simulink model "projekatSimulink"  (R2023b)
settings: Solver=VariableStepAuto  StartTime=0.0  StopTime=10.0  RelTol=1e-3
values from neighbouring files (symbols this model uses):
  A = [0 1 0 0 0; a21 a22 a23 a24 0; 0 0 0 1 0; a41 a42 a43 a44 a45; 0 0 0 a54 a55]    [projekatMatlab.m]
  a21 = k/(5*m)    (= 4000)    [projekatMatlab.m]
  a22 = b/(5*m)    (= 0.75)    [projekatMatlab.m]
  a23 = -k/(5*m)    (= -4000)    [projekatMatlab.m]
  a24 = -b/(5*m)    (= -0.75)    [projekatMatlab.m]
  a41 = -k/Mt    (= -61538.4615385)    [projekatMatlab.m]
  a42 = -b/Mt    (= -11.5384615385)    [projekatMatlab.m]
  a43 = k/Mt    (= 61538.4615385)    [projekatMatlab.m]
  a44 = -(Bp+b)/Mt    (= -13.8461538462)    [projekatMatlab.m]
  a45 = Ap/Mt    (= 0.000230769230769)    [projekatMatlab.m]
  a54 = -4*Be*Ap/Vt    (= -3900000000)    [projekatMatlab.m]
  a55 = -(Ctp+Kc)*4*Be/Vt    (= -2.6)    [projekatMatlab.m]
  b = 150    [projekatMatlab.m]
  B = [0; 0; 0; 0; b51]    [projekatMatlab.m]
  b51 = Kq*4*Be*Kt/(Vt*r*R*Kf)    (= 95766666.6667)    [projekatMatlab.m]
  C = [1 0 0 0 0]    [projekatMatlab.m]
  k = 8e5    (= 800000)    [projekatMatlab.m]
libraries: slpidlib x1
settings Model: Creator=Mi-Store  LastModifiedBy=Mi-Store

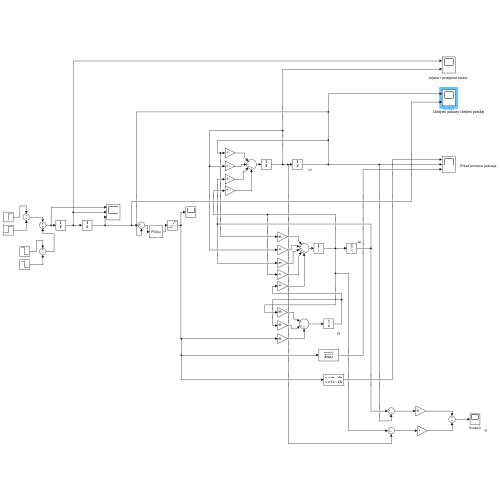
[thumbnail: Simulink's stored preview of the top-level diagram]
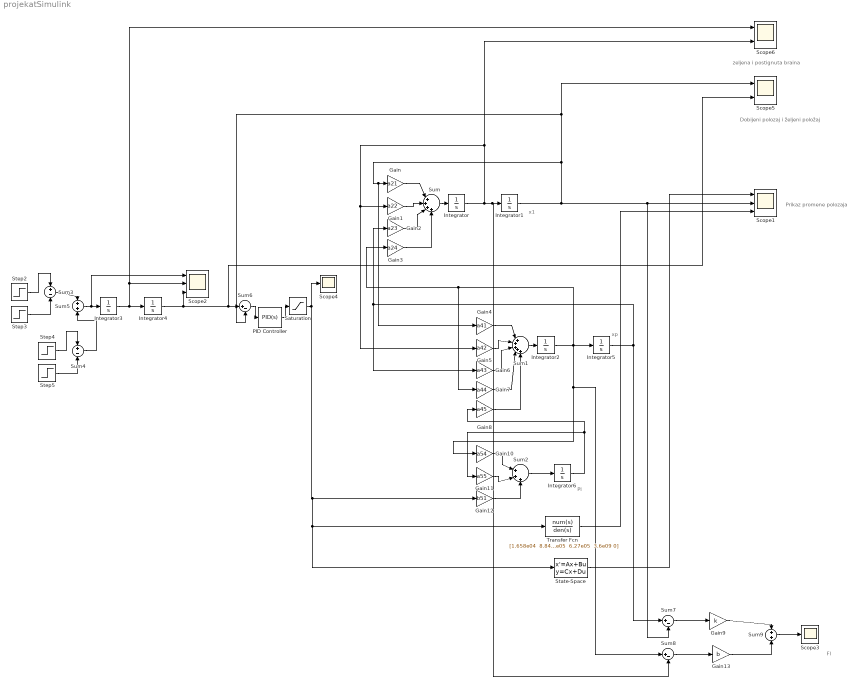
== system projekatSimulink ==
  note: zeljena i postignuta braina
  note: Dobijeni polozaj i željeni položaj
  note: Prikaz promene polozaja
  note: Fl
  note: Pl
  note: xp
  note: x1
  Gain : Gain  Gain=a21
  Gain1 : Gain  Gain=a22
  Gain10 : Gain  Gain=a54
  Gain11 : Gain  Gain=a55
  Gain12 : Gain  Gain=b51
  Gain13 : Gain  Gain=b
  Gain2 : Gain  Gain=a23
  Gain3 : Gain  Gain=a24
  Gain4 : Gain  Gain=a41
  Gain5 : Gain  Gain=a42
  Gain6 : Gain  Gain=a43
  Gain7 : Gain  Gain=a44
  Gain8 : Gain  Gain=a45
  Gain9 : Gain  Gain=k
  Integrator{,1..6} (7 alike) : Integrator
  PID Controller : slpidlib/PID Controller  Controller=PID  Form=Parallel  TimeDomain=Continuous-time  UseExternalTs=off  SampleTime=-1  IntegratorMethod=Forward Euler  FilterMethod=Forward Euler  ControllerParametersSource=internal  P=180  I=10  UseKiTs=on  D=0  N=100  UseFilter=on  TunerSelectOption=Transfer Function Based (PID Tuner App)  InitialConditionSource=internal  InitialConditionForIntegrator=0  InitialConditionForFilter=0  DifferentiatorICPrevScaledInput=0  ExternalReset=none  TrackingMode=off  Kt=1  LimitOutput=off  SatLimitsSource=internal  UpperSaturationLimit=inf  LowerSaturationLimit=-inf  LinearizeAsGain=on  AntiWindupMode=none  Kb=1  LimitIntegrator=off  UpperIntegratorSaturationLimit=inf  LowerIntegratorSaturationLimit=-inf  POutMin=[]  POutMax=[]  IOutMin=[]  IOutMax=[]  DOutMin=[]  DOutMax=[]  NOutMin=[]  NOutMax=[]  SumOutMin=[]  SumOutMax=[]  SaturationOutMin=[]  SaturationOutMax=[]  PParamMin=[]  PParamMax=[]  IParamMin=[]  IParamMax=[]  DParamMin=[]  DParamMax=[]  NParamMin=[]  NParamMax=[]  KbParamMin=[]  KbParamMax=[]  KtParamMin=[]  KtParamMax=[]  KbOutMin=[]  KbOutMax=[]  KtOutMin=[]  KtOutMax=[]  IntegratorOutMin=[]  IntegratorOutMax=[]  FilterOutMin=[]  FilterOutMax=[]  SumI1OutMin=[]  SumI1OutMax=[]  SumI2OutMin=[]  SumI2OutMax=[]  SumI3OutMin=[]  SumI3OutMax=[]  SumI4OutMin=[]  SumI4OutMax=[]  SumDOutMin=[]  SumDOutMax=[]  DifferentiatorOutMin=[]  DifferentiatorOutMax=[]  FilterDiffOutCoefMin=[]  FilterDiffOutCoefMax=[]  ReciprocalOutMin=[]  ReciprocalOutMax=[]  SumDenOutMin=[]  SumDenOutMax=[]  SumNumOutMin=[]  SumNumOutMax=[]  DivideOutMin=[]  DivideOutMax=[]  UdiffTsProdOutMin=[]  UdiffTsProdOutMax=[]  NTsProdOutMin=[]  NTsProdOutMax=[]  UintegralTsProdOutMin=[]  UintegralTsProdOutMax=[]  UngainTsProdOutMin=[]  UngainTsProdOutMax=[]  ClampingZeroOutDataTypeStr=Inherit: Inherit via back propagation  ClampingZeroOutMin=[]  ClampingZeroOutMax=[]  FilterDenConstantOutDataTypeStr=Inherit: Inherit via back propagation  FilterDenConstantOutMin=[]  FilterDenConstantOutMax=[]  PCopyOutDataTypeStr=Inherit: Inherit via back propagation  PCopyOutMin=[]  PCopyOutMax=[]  NCopyOutDataTypeStr=Inherit: Inherit via back propagation  NCopyOutMin=[]  NCopyOutMax=[]  IntegratorContinuousStateAttributes=''  IntegratorStateMustResolveToSignalObject=off  IntegratorRTWStateStorageClass=Auto  FilterContinuousStateAttributes=''  FilterStateMustResolveToSignalObject=off  FilterRTWStateStorageClass=Auto  ParallelPVariant=InternalParameters  IdealPVariant=Disabled  IVariant=InternalParameters  DVariant=InternalParameters  IntegratorVariant=Continuous  SatVariant=Disabled  AWVariant=Passthrough  PCopyVariant=Disabled  TRVariant=Disabled  FdbkBlocksVariant=Forward  IdealPFdbkVariant=Disabled  SatFdbkVariant=Disabled  DerivativeFilterVariant=ContFilter  NVariant=InternalParameters  NCopyVariant=Disabled  FilterICVariant=InternalICsFilter  IntegratorICVariant=InternalICs  ExternalResetVariant=Disabled  TRSumVariant=Passthrough  SumFdbkVariant=Disabled  SumVariant=Sum_PID  TsampFilterVariant=InternalTs  TsampNgainVariant=Passthrough  TsampIntegralVariant=Disabled_SignalSpec  ExternalSaturationOutDataTypeStr=Inherit: Same as second input
  Saturation : Saturate  UpperLimit=24  LowerLimit=0
  Scope1 : Scope  NumInputPorts=3
  Scope2 : Scope  NumInputPorts=3
  Scope3 : Scope
  Scope4 : Scope
  Scope5 : Scope  NumInputPorts=2
  Scope6 : Scope  NumInputPorts=2
  State-Space : StateSpace  A=A  B=B  C=C  D=0  InitialCondition=0
  Step2 : Step  Time=0  After=3.12  SampleTime=0
  Step3 : Step  Time=0.2  After=3.12  SampleTime=0
  Step4 : Step  Time=0.8  After=-3.12  SampleTime=0
  Step5 : Step  After=-3.12  SampleTime=0
  Sum : Sum  Inputs=|++++
  Sum1 : Sum  Inputs=|+++++
  Sum2 : Sum  Inputs=|+++
  Sum3 : Sum  Inputs=+-
  Sum4 : Sum  Inputs=+-
  Sum5 : Sum
  Sum6 : Sum  Inputs=|+-
  Sum7 : Sum  Inputs=|+-
  Sum8 : Sum  Inputs=|+-
  Sum9 : Sum
  Transfer Fcn : TransferFcn  Numerator="[1.658e04  8.84e07]"  Denominator="[17.2  8.425e05  6.27e05  3.6e09 0]"
  wires:
  Sum4/1 -> Sum5/2
  Sum5/1 -> Scope2/1, Integrator3/1
  Step3/1 -> Sum3/2
  Sum3/1 -> Sum5/1
  Integrator3/1 -> Scope6/1, Scope2/2, Integrator4/1
  Step4/1 -> Sum4/1
  Integrator4/1 -> Scope5/2, Sum6/1, Scope2/3
  Saturation/1 -> Scope4/1, State-Space/1, Transfer Fcn/1, Gain12/1
  Step5/1 -> Sum4/2
  Step2/1 -> Sum3/1
  Integrator/1 -> Sum8/2, Integrator1/1, Scope6/2, Gain5/1, Gain1/1
  Sum/1 -> Integrator/1
  Gain/1 -> Sum/1
  Gain1/1 -> Sum/2
  Gain2/1 -> Sum/3
  Gain3/1 -> Sum/4
  Integrator1/1 -> Gain4/1, Gain/1, Scope5/1, Sum6/2, Sum7/2, Scope1/2
  Integrator5/1 -> Sum7/1, Gain6/1, Gain2/1
  Gain5/1 -> Sum1/2
  Gain7/1 -> Sum1/4
  Gain6/1 -> Sum1/3
  Sum1/1 -> Integrator2/1
  Integrator2/1 -> Sum8/1, Gain10/1, Integrator5/1, Gain7/1, Gain3/1
  Gain4/1 -> Sum1/1
  Gain8/1 -> Sum1/5
  Gain12/1 -> Sum2/3
  Gain11/1 -> Sum2/2
  Gain10/1 -> Sum2/1
  Sum2/1 -> Integrator6/1
  Integrator6/1 -> Gain8/1, Gain11/1
  Transfer Fcn/1 -> Scope1/3
  State-Space/1 -> Scope1/1
  Sum6/1 -> PID Controller/1
  PID Controller/1 -> Saturation/1
  Sum7/1 -> Gain9/1
  Sum8/1 -> Gain13/1
  Gain9/1 -> Sum9/1
  Gain13/1 -> Sum9/2
  Sum9/1 -> Scope3/1
